simulink model "test"  (Simulink 9.0)
settings: Solver=ode45  StartTime=0.0  StopTime=10.0  RelTol=1e-3  EnableMultiTasking=on
undefined symbols (not defined in the file or in its folder): W1, W2, W3, W4
libraries: cstblocks x1
settings Model: Creator=gscorlet  LastModifiedBy=DEHAEZE
settings DataIOCC: LimitDataPoints=on  SignalLoggingSaveFormat=ModelDataLogs
settings OptimizationCC: BooleanDataType=off  DefaultParameterBehavior=Inlined  BufferReuse=off  ExpressionDepthLimit=2147483647  InitFltsAndDblsToZero=on
settings DebuggingCC: SaveWithParameterizedLinksMsg=none  SignalResolutionControl=TryResolveAllWithWarning  MultiTaskDSMMsg=warning  MultiTaskCondExecSysMsg=none  FcnCallInpInsideContextMsg=warning  StateNameClashWarn=warning  InitInArrayFormatMsg=none  StrictBusMsg=None
settings HardwareCC: TargetUnknown=on
settings GRTTargetCC: GeneratePreprocessorConditionals=Disable all  CombineOutputUpdateFcns=off  GRTInterface=on

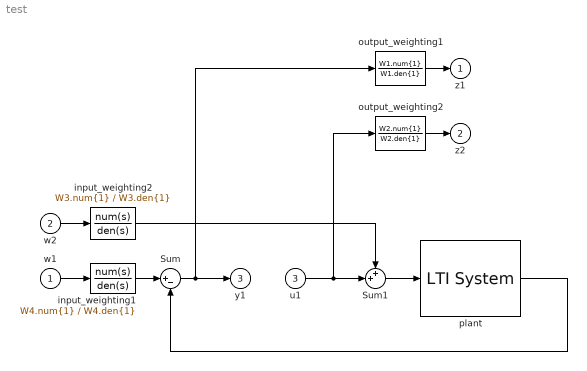
== system test ==
  w1 : Inport
  w2 : Inport  Port=2
  u1 : Inport  Port=3
  Sum : Sum  Inputs=|+-  SaturateOnIntegerOverflow=on  InputSameDT=on  OutDataTypeStr=Inherit: Same as first input
  Sum1 : Sum  Inputs=++|  SaturateOnIntegerOverflow=on  InputSameDT=on  OutDataTypeStr=Inherit: Same as first input
  input_weighting1 : TransferFcn  Numerator=W4.num{1}  Denominator=W4.den{1}
  input_weighting2 : TransferFcn  Numerator=W3.num{1}  Denominator=W3.den{1}
  output_weighting1 : TransferFcn  Numerator=W1.num{1}  Denominator=W1.den{1}
  output_weighting2 : TransferFcn  Numerator=W2.num{1}  Denominator=W2.den{1}
  plant : cstblocks/LTI System  sys=f_sys  IC=[]
  z1 : Outport  InitialOutput=0
  z2 : Outport  Port=2  InitialOutput=0
  y1 : Outport  Port=3  InitialOutput=0
  wires:
  output_weighting1/1 -> z1/1
  w1/1 -> input_weighting1/1
  Sum/1 -> y1/1, output_weighting1/1
  u1/1 -> Sum1/2, output_weighting2/1
  Sum1/1 -> plant/1
  plant/1 -> Sum/2
  input_weighting1/1 -> Sum/1
  output_weighting2/1 -> z2/1
  w2/1 -> input_weighting2/1
  input_weighting2/1 -> Sum1/1
